simulink model "EarCanal"  (R2024a)
settings: Solver=VariableStepAuto  StartTime=0.0  StopTime=T  RelTol=1e-3
model workspace (MAT data in the model file):
  C0_1 = Simulink.Parameter
  C0_1.Value = Simulink.data.Expression
  C0_1.Value.ExpressionString = "pi*a1^2*l1/(rho*c^2)"
  C0_1.Complexity = 'real'
  C0_1.Dimensions = -1
  C0_1.DataType = 'auto'
  C0_2 = Simulink.Parameter
  C0_2.Value = Simulink.data.Expression
  C0_2.Value.ExpressionString = "pi*a2^2*l2/(rho*c^2)"
  C0_2.Complexity = 'real'
  C0_2.Dimensions = -1
  C0_2.DataType = 'auto'
  C1_1 = Simulink.Parameter
  C1_1.Value = Simulink.data.Expression
  C1_1.Value.ExpressionString = "(gamma - 1)*C0_1"
  C1_1.Complexity = 'real'
  C1_1.Dimensions = -1
  C1_1.DataType = 'auto'
  C1_2 = Simulink.Parameter
  C1_2.Value = Simulink.data.Expression
  C1_2.Value.ExpressionString = "(gamma - 1)*C0_2"
  C1_2.Complexity = 'real'
  C1_2.Dimensions = -1
  C1_2.DataType = 'auto'
  Cp = Simulink.Parameter
  Cp.Value = 1010
  Cp.Complexity = 'real'
  Cp.Dimensions = [1 1]
  Cp.DataType = 'auto'
  L0_1 = Simulink.Parameter
  L0_1.Value = Simulink.data.Expression
  L0_1.Value.ExpressionString = "rho*l1/(pi*a1^2)"
  L0_1.Complexity = 'real'
  L0_1.Dimensions = -1
  L0_1.DataType = 'auto'
  L0_2 = Simulink.Parameter
  L0_2.Value = Simulink.data.Expression
  L0_2.Value.ExpressionString = "rho*l2/(pi*a2^2)"
  L0_2.Complexity = 'real'
  L0_2.Dimensions = -1
  L0_2.DataType = 'auto'
  Rt_1 = Simulink.Parameter
  Rt_1.Value = Simulink.data.Expression
  Rt_1.Value.ExpressionString = "rho^2*c^2*Cp/(8*pi*kappa*(gamma - 1)*l1)"
  Rt_1.Complexity = 'real'
  Rt_1.Dimensions = -1
  Rt_1.DataType = 'auto'
  Rt_2 = Simulink.Parameter
  Rt_2.Value = Simulink.data.Expression
  Rt_2.Value.ExpressionString = "rho^2*c^2*Cp/(8*pi*kappa*(gamma - 1)*l2)"
  Rt_2.Complexity = 'real'
  Rt_2.Dimensions = -1
  Rt_2.DataType = 'auto'
  Rv_1 = Simulink.Parameter
  Rv_1.Value = Simulink.data.Expression
  Rv_1.Value.ExpressionString = "8*pi*rho*nu*l1/(pi*a1^2)^2"
  Rv_1.Complexity = 'real'
  Rv_1.Dimensions = -1
  Rv_1.DataType = 'auto'
  Rv_2 = Simulink.Parameter
  Rv_2.Value = Simulink.data.Expression
  Rv_2.Value.ExpressionString = "8*pi*rho*nu*l2/(pi*a2^2)^2"
  Rv_2.Complexity = 'real'
  Rv_2.Dimensions = -1
  Rv_2.DataType = 'auto'
  T = Simulink.Parameter
  T.Value = 3
  T.Complexity = 'real'
  T.Dimensions = [1 1]
  T.Description = 'simulation time '
  T.DataType = 'auto'
  a1 = Simulink.Parameter
  a1.Value = 0.005
  a1.Complexity = 'real'
  a1.Dimensions = [1 1]
  a1.DataType = 'auto'
  a2 = Simulink.Parameter
  a2.Value = 0.0035
  a2.Complexity = 'real'
  a2.Dimensions = [1 1]
  a2.DataType = 'auto'
  c = Simulink.Parameter
  c.Value = 343
  c.Complexity = 'real'
  c.Dimensions = [1 1]
  c.DataType = 'auto'
  dt = Simulink.Parameter
  dt.Value = 2.26757369615e-05
  dt.Complexity = 'real'
  dt.Dimensions = [1 1]
  dt.Description = 'sampling time '
  dt.DataType = 'auto'
  gamma = Simulink.Parameter
  gamma.Value = 1.4
  gamma.Complexity = 'real'
  gamma.Dimensions = [1 1]
  gamma.DataType = 'auto'
  kappa = Simulink.Parameter
  kappa.Value = 0.0257
  kappa.Complexity = 'real'
  kappa.Dimensions = [1 1]
  kappa.DataType = 'auto'
  l1 = Simulink.Parameter
  l1.Value = 0.003
  l1.Complexity = 'real'
  l1.Dimensions = [1 1]
  l1.DataType = 'auto'
  l2 = Simulink.Parameter
  l2.Value = 0.0095
  l2.Complexity = 'real'
  l2.Dimensions = [1 1]
  l2.DataType = 'auto'
  nu = Simulink.Parameter
  nu.Value = 1.568e-05
  nu.Complexity = 'real'
  nu.Dimensions = [1 1]
  nu.DataType = 'auto'
  rho = Simulink.Parameter
  rho.Value = 1.21
  rho.Complexity = 'real'
  rho.Dimensions = [1 1]
  rho.DataType = 'auto'
undefined symbols (not defined in the file): acoustic
libraries: acoustic_lib x5, nesl_utility x4, simulink x1
settings Model: Creator=andychen  LastModifiedBy=ftiong
settings DataIOCC: OutputOption=SpecifiedOutputTimes  OutputTimes=0:dt:T

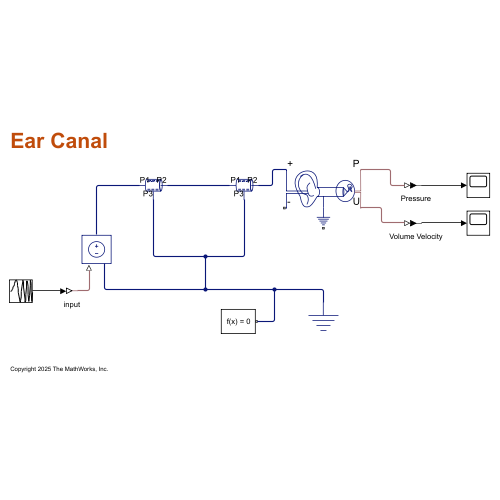
[thumbnail: Simulink's stored preview of the top-level diagram]
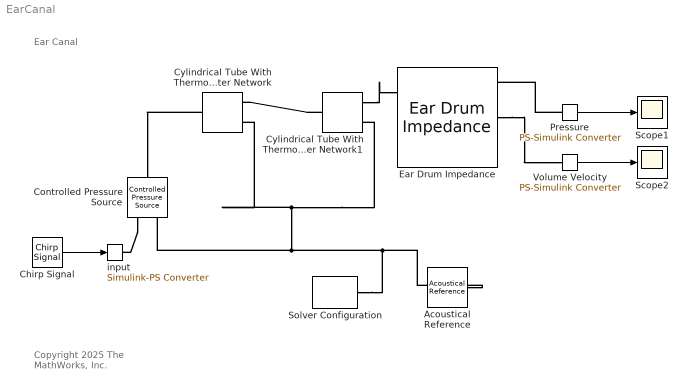
== system EarCanal ==
  note: Ear Canal
  note: Copyright 2025 The MathWorks, Inc.
  Acoustical Reference : acoustic_lib/Acoustical Elements/Acoustical Reference
      settings: SourceProductName=Acoustic  InternalSimscapePortConfiguration="{\"Bottom\":[],\"Left\":[],\"Right\":[],\"Top\":[{\"id\":\"pp\",\"label\":\"\",\"type\":\"acoustic.acoustic\"}]}"
  Chirp Signal : simulink/Sources/Chirp Signal  f1=10  T=T  f2=20e3
  Controlled Pressure Source : acoustic_lib/Acoustical Sources/Controlled Pressure Source
      settings: SourceProductName=Acoustic  InternalSimscapePortConfiguration="{\"Bottom\":[],\"Left\":[{\"id\":\"pp\",\"label\":\"\",\"type\":\"acoustic.acoustic\"}],\"Right\":[{\"id\":\"pT\",\"label\":\"\",\"type\":\"input\"},{\"id\":\"nn\",\"label\":\"\",\"type\":\"acoustic.acoustic\"}],\"Top\":[]}"
  Cylindrical Tube With Thermoviscous Losses Using Foster Network : acoustic_lib/Applications/Tubes and Horns/Cylindrical Tube With Thermoviscous Losses Using Foster Network  a=a1 m  length=l1 m  mdl=acoustic.enum.Tubemdl.simple  order=4  Ndl=20
      settings: SourceProductName=Acoustic  InternalSimscapePortConfiguration="{\"Bottom\":[{\"id\":\"p3\",\"label\":\"P3\",\"type\":\"acoustic.acoustic\"}],\"Left\":[{\"id\":\"p1\",\"label\":\"P1\",\"type\":\"acoustic.acoustic\"}],\"Right\":[{\"id\":\"p2\",\"label\":\"P2\",\"type\":\"acoustic.acoustic\"}],\"Top\":[]}"
  Cylindrical Tube With Thermoviscous Losses Using Foster Network1 : acoustic_lib/Applications/Tubes and Horns/Cylindrical Tube With Thermoviscous Losses Using Foster Network  a=a2 m  length=l2 m  mdl=acoustic.enum.Tubemdl.simple  order=4  Ndl=20
      settings: SourceProductName=Acoustic  InternalSimscapePortConfiguration="{\"Bottom\":[{\"id\":\"p3\",\"label\":\"P3\",\"type\":\"acoustic.acoustic\"}],\"Left\":[{\"id\":\"p1\",\"label\":\"P1\",\"type\":\"acoustic.acoustic\"}],\"Right\":[{\"id\":\"p2\",\"label\":\"P2\",\"type\":\"acoustic.acoustic\"}],\"Top\":[]}"
  Ear Drum Impedance : acoustic_lib/Applications/Human Ear/Ear Drum Impedance  Ma1=82.9 Pa*s^2/m^3  Ma2=9400 Pa*s^2/m^3  Ma3=130.3 Pa*s^2/m^3  Ma4=983.8 Pa*s^2/m^3  Ma5=133.4 Pa*s^2/m^3  Ca1=0.7e-12 m^3/Pa  Ca2=2.34e-12 m^3/Pa  Ca3=1.5e-12 m^3/Pa  Ca4=2.73e-12 m^3/Pa  Ca5=1.517e-12 m^3/Pa  Ra2=55.66e6 Pa*s/m^3  Ra4=27.99e6 Pa*s/m^3  damping1=acoustic.enum.R1(1)  damping3=acoustic.enum.R3(1)  damping5=acoustic.enum.R5(1)  Ra1=4.22e5 Pa*s/m^3  Ra3=4.22e5 Pa*s/m^3  Ra5=3.22e6 Pa*s/m^3
      settings: SourceProductName=Acoustic  InternalSimscapePortConfiguration="{\"Bottom\":[{\"id\":\"ca\",\"label\":\"\",\"type\":\"acoustic.acoustic\"}],\"Left\":[{\"id\":\"pa\",\"label\":\"+\",\"type\":\"acoustic.acoustic\"},{\"id\":\"na\",\"label\":\"-\",\"type\":\"acoustic.acoustic\"}],\"Right\":[{\"id\":\"P\",\"label\":\"P\",\"type\":\"output\"},{\"id\":\"U\",\"label\":\"U\",\"type\":\"output\"}],\"Top\":[]}"
  Pressure : nesl_utility/PS-Simulink Converter  PhysicalDomain=network_engine_domain  SubClassName=ps_output  LeftPortType=input  RightPortType=output  PseudoPeriodic=off  Frequencies=[]  VectorFormat=inherit  Unit=inherit  AffineConversion=off
  Scope1 : Scope
  Scope2 : Scope
  Solver Configuration : nesl_utility/Solver Configuration  PhysicalDomain=network_engine_domain  SubClassName=solver  LeftPortType=input  RightPortType=generic  Tones=[]  Harmonics=[]  SimulateNoise=off  Profile=off  UseLocalSampling=off  EnableSwitchedLinearOptims=on  FrequencyDomain=off  UseCCode=off  RelTol=0.001  AbsTol=0.001  MinStep=1e-09  ToWorkspace=off  RevertToSquareIcSolve=off  NumHomotopyIterations=100  PhasorMode=off  PhasorModeNumHarmonics=1  ConsistencySolver=NEWTON_XTOL_AFTER_FTOL  IndexReductionMethod=DerivativeReplacement  DoDC=off  ResidualTolerance=1e-09  ConsistencyTolSource=GLOBAL  ConsistencyAbsTol=0.001  ConsistencyRelTol=0.001  ConsistencyTolFactor=0.001  UseLocalSolver=off  LocalSolverChoice=NE_BACKWARD_EULER_ADVANCER  ResolveIndetEquations=on  FunctionEvalNumThread=1  LocalSolverSampleTime=0.001  DoFixedCost=off  MaxNonlinIter=3  MaxModeIter=2  ComputeImpulses=off  ImpulseIterations=2  LinearAlgebra=auto  LinearAlgebraNumThread=0  EquationFormulation=NE_TIME_EF  DelaysMemoryBudget=1024  AutomaticFiltering=on  FilteringTimeConstant=0.001  PartitionStorageMethod=AS_NEEDED  PartitionMemoryBudget=1024  PartitionMethod=ROBUST  MultibodyUseLocalSolver=off  MultibodyLocalSolverChoice=ODE1  MultibodyLocalSolverSampleTime=0.001
  Volume Velocity : nesl_utility/PS-Simulink Converter  PhysicalDomain=network_engine_domain  SubClassName=ps_output  LeftPortType=input  RightPortType=output  PseudoPeriodic=off  Frequencies=[]  VectorFormat=inherit  Unit=inherit  AffineConversion=off
  input : nesl_utility/Simulink-PS Converter  PhysicalDomain=network_engine_domain  SubClassName=ps_input  LeftPortType=input  RightPortType=output  PseudoPeriodic=off  Frequencies=[]  NoiseDistribution=none  NoiseParameters=[]  Unit=1  AffineConversion=off  FilteringAndDerivatives=provide  SimscapeFilterOrder=1  InputFilterTimeConstant=0.001  UdotUserProvided=0
  wires:
  Chirp Signal/1 -> input/1
  Pressure/1 -> Scope1/1
  Volume Velocity/1 -> Scope2/1
  connections:
  Controlled Pressure Source/RConn1 -- input/RConn1
  Ear Drum Impedance/RConn2 -- Volume Velocity/LConn1
  Cylindrical Tube With Thermoviscous Losses Using Foster Network1/LConn1 -- Cylindrical Tube With Thermoviscous Losses Using Foster Network/RConn1
  Cylindrical Tube With Thermoviscous Losses Using Foster Network1/RConn2 -- Cylindrical Tube With Thermoviscous Losses Using Foster Network/RConn2 -- Solver Configuration/RConn1 -- Acoustical Reference/LConn1 -- Controlled Pressure Source/RConn2
  Cylindrical Tube With Thermoviscous Losses Using Foster Network1/RConn1 -- Ear Drum Impedance/LConn1
  Cylindrical Tube With Thermoviscous Losses Using Foster Network/LConn1 -- Controlled Pressure Source/LConn1
  Pressure/LConn1 -- Ear Drum Impedance/RConn1
